simulink model "lab02_3_2b"  (R2013a)
settings: Solver=ode45  StartTime=0.0  StopTime=3  RelTol=1e-3
values from neighbouring files (symbols this model uses):
  A1 = 4    [Lab02.m]
  A2 = 20    [Lab02.m]
  Bt = 0.005    [Lab02.m]
  Jt = 0.05    [Lab02.m]
  kc = 0.5    [Lab02.m]
  kg = 5    [Lab02.m]
  kpre = 0.2423076923    [Lab02.m]
  kt = 0.25    [Lab02.m]
  kw = 0.5    [Lab02.m]
  Lf = 0    [Lab02.m]
  Lg = 0    [Lab02.m]
  Lm = 0    [Lab02.m]
  Rf = 50    [Lab02.m]
  Rg = 1    [Lab02.m]
  Rm = 1    [Lab02.m]
settings Model: Creator=ansanf  LastModifiedBy=ToniO
settings DataIOCC: SignalLoggingSaveFormat=ModelDataLogs
settings DebuggingCC: MultiTaskDSMMsg=warning  MultiTaskCondExecSysMsg=none  StateNameClashWarn=none  StrictBusMsg=None
settings RTWCC: IncludeERTFirstTime=on

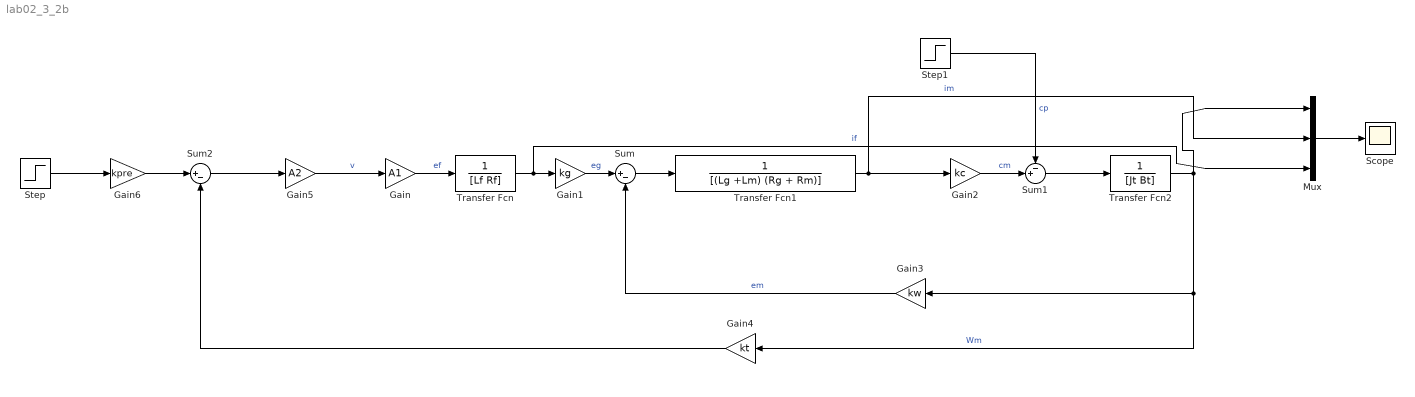
== system lab02_3_2b ==
  Gain : Gain  Gain=A1
  Gain1 : Gain  Gain=kg
  Gain2 : Gain  Gain=kc
  Gain3 : Gain  Gain=kw
  Gain4 : Gain  Gain=kt
  Gain5 : Gain  Gain=A2
  Gain6 : Gain  Gain=kpre
  Mux : Mux  Inputs=3
  Scope : Scope
      settings: SaveName=ScopeData3_2
  Step : Step  Time=0  After=100  SampleTime=0
  Step1 : Step  Time=5  SampleTime=0
  Sum : Sum  Inputs=|+-
  Sum1 : Sum  Inputs=-+|
  Sum2 : Sum  Inputs=|+-
  Transfer Fcn : TransferFcn  Denominator=[Lf Rf]
  Transfer Fcn1 : TransferFcn  Denominator=[(Lg +Lm) (Rg + Rm)]
  Transfer Fcn2 : TransferFcn  Denominator=[Jt Bt]
  wires:
  Gain/1 -> Transfer Fcn/1  "ef"
  Sum/1 -> Transfer Fcn1/1
  Transfer Fcn1/1 -> Mux/2, Gain2/1  "im"
  Transfer Fcn/1 -> Mux/3, Gain1/1  "if"
  Transfer Fcn2/1 -> Gain4/1, Gain3/1, Mux/1  "Wm"
  Step1/1 -> Sum1/1  "cp"
  Sum1/1 -> Transfer Fcn2/1
  Gain2/1 -> Sum1/2  "cm"
  Gain1/1 -> Sum/1  "eg"
  Gain3/1 -> Sum/2  "em"
  Mux/1 -> Scope/1
  Gain6/1 -> Sum2/1
  Sum2/1 -> Gain5/1
  Gain4/1 -> Sum2/2
  Gain5/1 -> Gain/1  "v"
  Step/1 -> Gain6/1
